simulink model "Virtual_Engine_Airpath_Model_PRT"  (R2016b)
settings: Solver=FixedStepDiscrete  StartTime=0  StopTime=inf  RelTol=1e-3  SampleTimeConstraint=STIndependent  EnableMultiTasking=on
InitFcn:
  | % Call parameters initialization function
  | % run optiTruck_init_sim.m;
StopFcn:
  | %optiTruck_post_sim;
  | %optiTruck_plot_sim;
settings Model: Creator=engin  LastModifiedBy=bunver
settings DataIOCC: SaveFormat=StructureWithTime  SaveOutput=off  DSMLogging=off  VisualizeSimOutput=off  SaveTime=off  SignalLoggingName=Results
settings OptimizationCC: BlockReduction=off  ConditionallyExecuteInputs=off  LifeSpan=inf
settings DebuggingCC: AllowSymbolicDim=off  SFUnexpectedBacktrackingDiag=warning  SFNoUnconditionalDefaultTransitionDiag=warning  SFExecutionAtInitializationDiag=none
settings ModelReferenceCC: ModelReferenceNumInstancesAllowed=Single  PropagateSignalLabelsOutOfModel=off
settings GRTTargetCC: TargetLangStandard=C89/C90 (ANSI)
settings ConfigComp: CovMetricSettings=dw  CovHtmlReporting=on  CovSaveCumulativeToWorkspaceVar=on  CovSaveSingleToWorkspaceVar=on  CovExternalEMLEnable=off

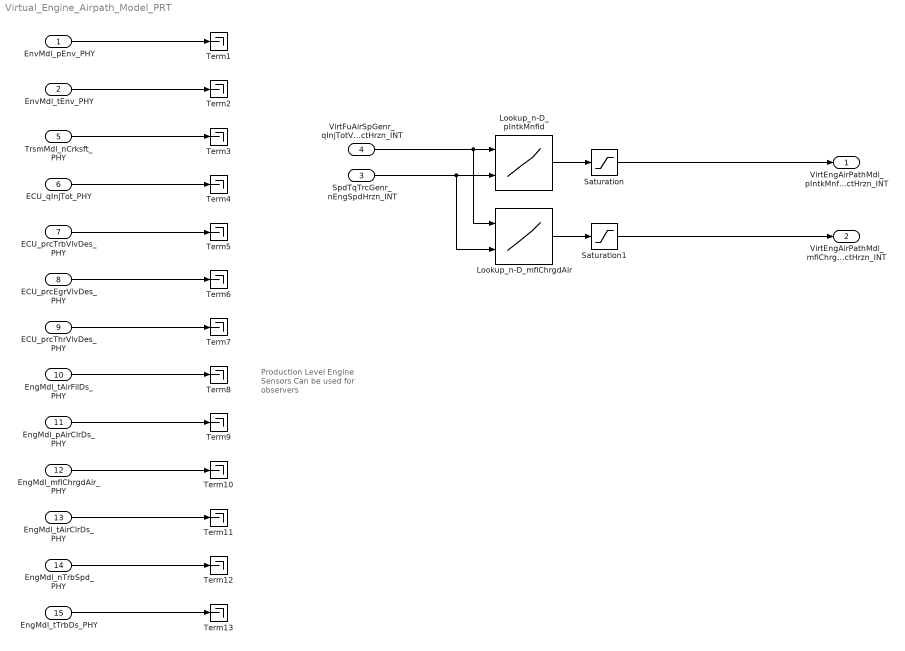
== system Virtual_Engine_Airpath_Model_PRT ==
  note: Production Level
      | Engine Sensors
      |
      | Can be used for observers
  EnvMdl_pEnv_PHY : Inport  OutDataTypeStr=double  PortDimensions=1
  EnvMdl_tEnv_PHY : Inport  Port=2  OutDataTypeStr=double  PortDimensions=1
  SpdTqTrcGenr_nEngSpdHrzn_INT : Inport  Port=3  PortDimensions=[400, 1]
  VirtFuAirSpGenr_qInjTotVectHrzn_INT : Inport  Port=4  PortDimensions=[400, 1]
  TrsmMdl_nCrksft_PHY : Inport  Port=5  OutDataTypeStr=double  PortDimensions=1
  ECU_qInjTot_PHY : Inport  Port=6  OutDataTypeStr=double  PortDimensions=1
  ECU_prcTrbVlvDes_PHY : Inport  Port=7  OutDataTypeStr=double  PortDimensions=1
  ECU_prcEgrVlvDes_PHY : Inport  Port=8  OutDataTypeStr=double  PortDimensions=1
  ECU_prcThrVlvDes_PHY : Inport  Port=9  OutDataTypeStr=double  PortDimensions=1
  EngMdl_tAirFilDs_PHY : Inport  Port=10  OutDataTypeStr=double  PortDimensions=1
  EngMdl_pAirClrDs_PHY : Inport  Port=11  OutDataTypeStr=double  PortDimensions=1
  EngMdl_mflChrgdAir_PHY : Inport  Port=12  OutDataTypeStr=double  PortDimensions=1
  EngMdl_tAirClrDs_PHY : Inport  Port=13  OutDataTypeStr=double  PortDimensions=1
  EngMdl_nTrbSpd_PHY : Inport  Port=14  OutDataTypeStr=double  PortDimensions=1
  EngMdl_tTrbDs_PHY : Inport  Port=15  OutDataTypeStr=double  PortDimensions=1
  Lookup_n-D_mflChrgdAir : Lookup_n-D  BreakpointsForDimension1=|  BreakpointsForDimension2=[0 550 600 700 800 900 1050 1200 1350 1500 1650 1800 1950 2100 2250 2400]  Table=[0 90 110 151 193 235 292 346 407 490 595 655 764 983 1207 1452;0 99 119 159 200 241 296 352 416 495 597 640 727 958 1192 1436;0 108 128 168 207 246 300 357 425 501 598 624 692 932 1177 1420;0 117 137 176 215 251 304 362 434 508 596 609 659 909 1163 1404;0 125 145 185 222 255 308 367 444 517 591 596 628 893 1149 1387;0 134 154 195 230 260 313 373 455 527 587 588 601 883 1137 1370;0 169 192 239 284 331 403 483 556 611 672 778 805 966 1103 1262;0 215 236 276 319 372 452 534 589 689 789 907 860 921 1051 1183;0 217 242 292 351 412 499 580 669 779 886 965 1021 1076 1108 1147;0 227 261 331 389 458 570 667 767 884 985 1066 1111 1148 1159 1165;0 252 289 365 423 507 641 760 880 994 1060 1130 1231 1202 1212 1226;0 307 339 402 451 525 691 858 977 1071 1198 1307 1348 1342 1337 1338;0 344 384 467 557 616 772 934 1057 1205 1310 1381 1422 1454 1477 1495;0 422 470 567 659 709 848 1027 1194 1297 1375 1442 1500 1500 1500 1500;0 486 530 617 703 792 1023 1148 1216 1365 1496 1500 1500 1500 1500 1500;0 539 596 712 829 946 1114 1246 1329 1385 1499 1500 1500 1500 1500 1500]/3600  ExtrapMethod=Clip  UseLastTableValue=on  RndMeth=Simplest  InputSameDT=on
      | [0
      | 5
      | 10
      | 15
      | 20
      | 25
      | 50
      | 75
      | 100
      | 125
      | 150
      | 175
      | 200
      | 230
      | 260
      | 290]'
  Lookup_n-D_pIntkMnfld : Lookup_n-D  BreakpointsForDimension1=|  BreakpointsForDimension2=[0 550 600 700 800 900 1050 1200 1350 1500 1650 1800 1950 2100 2250 2400]  Table=[923 1018 1029 1050 1071 1088 1093 1086 1135 1338 1476 1400 1351 1391 1442 1489;912 1025 1037 1061 1084 1104 1119 1117 1153 1346 1484 1416 1360 1392 1423 1449;900 1033 1046 1072 1097 1120 1145 1149 1174 1354 1490 1432 1370 1393 1404 1410;889 1040 1055 1084 1110 1136 1170 1180 1199 1361 1489 1452 1382 1394 1385 1371;878 1047 1063 1095 1124 1151 1194 1210 1227 1367 1483 1473 1398 1395 1365 1331;866 1055 1072 1107 1138 1166 1218 1241 1256 1374 1476 1495 1416 1396 1345 1292;808 1097 1125 1181 1243 1310 1373 1422 1419 1473 1546 1614 1487 1344 1226 1114;742 1191 1224 1285 1338 1424 1443 1494 1543 1608 1670 1719 1632 1371 1201 1060;663 1231 1284 1394 1465 1509 1555 1663 1705 1780 1875 1904 1788 1539 1357 1189;571 1312 1386 1537 1632 1738 1839 1918 1975 2008 2103 2067 1988 1870 1667 1455;500 1412 1485 1630 1737 1928 2110 2191 2201 2250 2336 2297 2356 2132 1952 1764;500 1521 1606 1771 1918 2034 2303 2402 2381 2495 2544 2488 2609 2468 2263 2057;500 1506 1638 1906 2197 2301 2512 2659 2677 2727 2756 2710 2657 2570 2445 2302;500 1495 1646 1949 2252 2532 2771 2779 2875 2901 3014 2905 2723 2629 2559 2491;500 1493 1644 1948 2267 2616 3058 3030 3039 3174 3223 3067 2921 2804 2711 2630;500 1586 1741 2049 2348 2629 2986 3209 3305 3264 3230 3174 3095 2998 2894 2786]*1e2  ExtrapMethod=Clip  UseLastTableValue=on  RndMeth=Simplest  InputSameDT=on
      | [0
      | 5
      | 10
      | 15
      | 20
      | 25
      | 50
      | 75
      | 100
      | 125
      | 150
      | 175
      | 200
      | 230
      | 260
      | 290]'
  Saturation : Saturate  UpperLimit=5000*1e2  LowerLimit=500*1e2
  Saturation1 : Saturate  UpperLimit=2000/3600  LowerLimit=0
  Term{1..13} (13 alike) : Terminator
  VirtEngAirPathMdl_pIntkMnfldVectHrzn_INT : Outport  OutDataTypeStr=double
  VirtEngAirPathMdl_mflChrgdAirVectHrzn_INT : Outport  Port=2  OutDataTypeStr=double
  wires:
  EngMdl_tTrbDs_PHY/1 -> Term13/1
  EngMdl_tAirClrDs_PHY/1 -> Term11/1
  ECU_prcThrVlvDes_PHY/1 -> Term7/1
  ECU_prcTrbVlvDes_PHY/1 -> Term5/1
  ECU_prcEgrVlvDes_PHY/1 -> Term6/1
  EnvMdl_tEnv_PHY/1 -> Term2/1
  EnvMdl_pEnv_PHY/1 -> Term1/1
  EngMdl_tAirFilDs_PHY/1 -> Term8/1
  EngMdl_nTrbSpd_PHY/1 -> Term12/1
  EngMdl_mflChrgdAir_PHY/1 -> Term10/1
  EngMdl_pAirClrDs_PHY/1 -> Term9/1
  Saturation/1 -> VirtEngAirPathMdl_pIntkMnfldVectHrzn_INT/1
  Saturation1/1 -> VirtEngAirPathMdl_mflChrgdAirVectHrzn_INT/1
  Lookup_n-D_pIntkMnfld/1 -> Saturation/1
  Lookup_n-D_mflChrgdAir/1 -> Saturation1/1
  SpdTqTrcGenr_nEngSpdHrzn_INT/1 -> Lookup_n-D_pIntkMnfld/2, Lookup_n-D_mflChrgdAir/2
  VirtFuAirSpGenr_qInjTotVectHrzn_INT/1 -> Lookup_n-D_mflChrgdAir/1, Lookup_n-D_pIntkMnfld/1
  TrsmMdl_nCrksft_PHY/1 -> Term3/1
  ECU_qInjTot_PHY/1 -> Term4/1
